simulink model "LQGdesign"  (R2019b)
settings: Solver=VariableStepAuto  StartTime=0.0  StopTime=3  RelTol=1e-3
values from neighbouring files (symbols this model uses):
  F2 = a*mass*g/(a+b)    (= 14.8072837402)    [main.m]
  g = 9.8    [EOM.m]    (also in main.m = 9.81)
  h0 = geometry_parameters(3)    [CalculateLoadCapacity.m]    (also in initialiseradialgap.m; main.m = 5e-05)
  Klqgi = lqr(Aaug,Baug,Qaug,Raug)    [main.m]
  Kps = (Vmax-Vmin)/(Hmax-Hmin)    (= 1666.66666667)    [main.m]
  Ksv = 30    [main.m]
  syskfd = c2d(syskf,Ts)    [main.m]
  tau = 0.12    [main.m]
  taus = 0.00125    [main.m]
  Ts = 1/fs    (= 0.001)    [main.m]
  xeq = x(end,1)    [main.m]
  yeq = x(end,3)    [main.m]
undefined symbols (not defined in the file or in its folder): DiscIntNeverNeededParam
libraries: neural x106, simulink x2
(part 1 of 3)
settings Model: Creator=Alexander  LastModifiedBy=Alexander

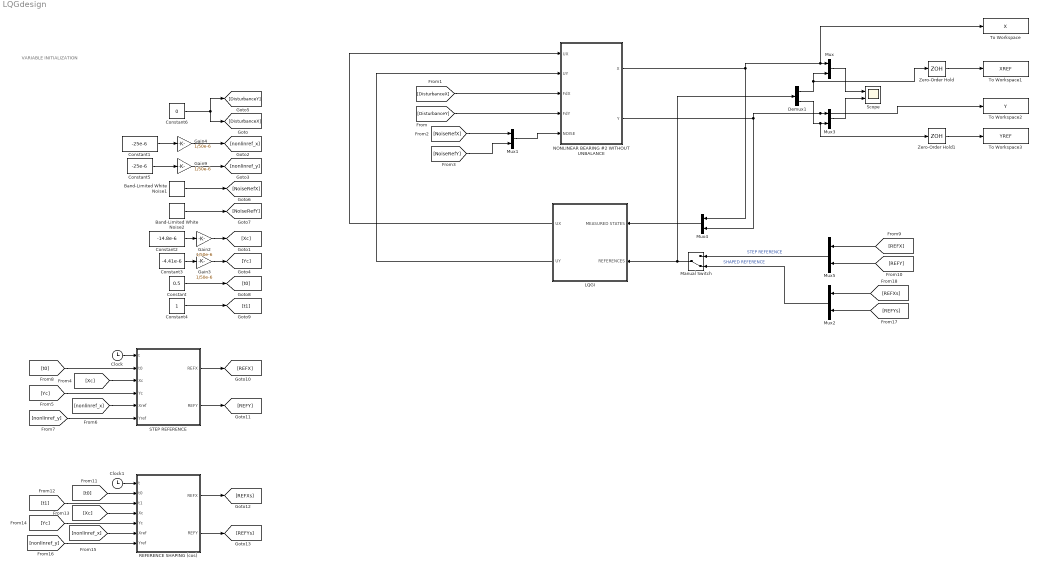
== system LQGdesign ==
  note: VARIABLE INITIALIZATION
  Band-Limited White Noise1 : simulink/Sources/Band-Limited White Noise  Cov=n_pow  Ts=Ts  seed=[23341]
  Band-Limited White Noise2 : simulink/Sources/Band-Limited White Noise  Cov=n_pow  Ts=1.1*Ts  seed=[23341]
  Clock : Clock
  Clock1 : Clock
  Constant : Constant  Value=0.5
  Constant1 : Constant  Value=-25e-6
  Constant2 : Constant  Value=-14.8e-6
  Constant3 : Constant  Value=-4.41e-6
  Constant4 : Constant
  Constant5 : Constant  Value=-25e-6
  Constant6 : Constant  Value=0
  Demux1 : Demux  Outputs=2
  Gain{2..4,9} (4 alike) : Gain  Gain=1/50e-6
  LQGI : Subsystem
  Manual Switch : ManualSwitch  CurrentSetting=0
  Mux{,1..5} (6 alike) : Mux  Inputs=2
  NONLINEAR BEARING #2 WITHOUT UNBALANCE : Subsystem
  REFERENCE SHAPING (cos) : MATLAB Function  TreatAsAtomicUnit=on
  STEP REFERENCE : MATLAB Function  TreatAsAtomicUnit=on
  Scope : Scope  NumInputPorts=2
  To Workspace : ToWorkspace  VariableName=X  SampleTime=-1
      settings: Save2DSignal=2-D array (concatenate along first dimension)
  To Workspace1 : ToWorkspace  VariableName=XREF  SampleTime=-1
      settings: Save2DSignal=2-D array (concatenate along first dimension)
  To Workspace2 : ToWorkspace  VariableName=Y  SampleTime=-1
      settings: Save2DSignal=2-D array (concatenate along first dimension)
  To Workspace3 : ToWorkspace  VariableName=YREF  SampleTime=-1
      settings: Save2DSignal=2-D array (concatenate along first dimension)
  Zero-Order Hold : ZeroOrderHold  SampleTime=Ts
  Zero-Order Hold1 : ZeroOrderHold  SampleTime=Ts
  wires:
  [nonlinref_x] -> STEP REFERENCE/5(Xref)
  Constant4/1 -> [t1]
  [NoiseRefY] -> Mux1/2
  Constant/1 -> [t0]
  [t0] -> STEP REFERENCE/2(t0)
  Clock/1 -> STEP REFERENCE/1(t)
  NONLINEAR BEARING #2 WITHOUT UNBALANCE/1(X) -> To Workspace/1, Mux/1, Mux4/1
  STEP REFERENCE/2(REFY) -> [REFY]
  Gain9/1 -> [nonlinref_y]
  Constant3/1 -> Gain3/1
  [Xc] -> STEP REFERENCE/3(Xc)
  [DisturbanceY] -> NONLINEAR BEARING #2 WITHOUT UNBALANCE/4(FdY)
  Mux3/1 -> Scope/2
  Gain3/1 -> [Yc]
  Gain2/1 -> [Xc]
  [DisturbanceX] -> NONLINEAR BEARING #2 WITHOUT UNBALANCE/3(FdX)
  NONLINEAR BEARING #2 WITHOUT UNBALANCE/2(Y) -> To Workspace2/1, Mux3/1, Mux4/2
  Constant5/1 -> Gain9/1
  STEP REFERENCE/1(REFX) -> [REFX]
  Demux1/1 -> Mux/2, Zero-Order Hold/1
  Gain4/1 -> [nonlinref_x]
  Mux2/1 -> Manual Switch/2  "SHAPED REFERENCE"
  REFERENCE SHAPING (cos)/1(REFX) -> [REFXs]
  Mux5/1 -> Manual Switch/1  "STEP REFERENCE"
  [Yc] -> STEP REFERENCE/4(Yc)
  [REFY] -> Mux5/2
  [REFXs] -> Mux2/1
  Mux/1 -> Scope/1
  [REFX] -> Mux5/1
  Constant2/1 -> Gain2/1
  [REFYs] -> Mux2/2
  Band-Limited White Noise1/1 -> [NoiseRefX]
  Demux1/2 -> Zero-Order Hold1/1, Mux3/2
  Mux1/1 -> NONLINEAR BEARING #2 WITHOUT UNBALANCE/5(NOISE)
  Clock1/1 -> REFERENCE SHAPING (cos)/1(t)
  [nonlinref_y] -> STEP REFERENCE/6(Yref)
  [nonlinref_x] -> REFERENCE SHAPING (cos)/6(Xref)
  Band-Limited White Noise2/1 -> [NoiseRefY]
  REFERENCE SHAPING (cos)/2(REFY) -> [REFYs]
  [Yc] -> REFERENCE SHAPING (cos)/5(Yc)
  [nonlinref_y] -> REFERENCE SHAPING (cos)/7(Yref)
  [Xc] -> REFERENCE SHAPING (cos)/4(Xc)
  Constant1/1 -> Gain4/1
  [t0] -> REFERENCE SHAPING (cos)/2(t0)
  [t1] -> REFERENCE SHAPING (cos)/3(t1)
  [NoiseRefX] -> Mux1/1
  Zero-Order Hold/1 -> To Workspace1/1
  Zero-Order Hold1/1 -> To Workspace3/1
  Constant6/1 -> [DisturbanceX], [DisturbanceY]
  Manual Switch/1 -> Demux1/1, LQGI/2(REFERENCES)
  LQGI/2("UY ") -> NONLINEAR BEARING #2 WITHOUT UNBALANCE/2(UY)
  LQGI/1(UX) -> NONLINEAR BEARING #2 WITHOUT UNBALANCE/1(UX)
  Mux4/1 -> LQGI/1(MEASURED STATES)

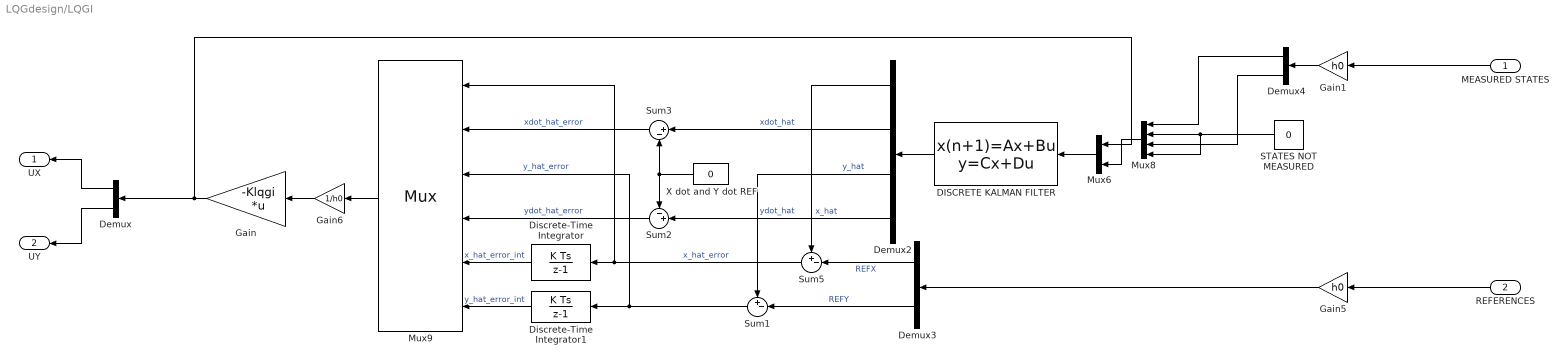
== system LQGdesign/LQGI ==
  MEASURED STATES : Inport
  REFERENCES : Inport  Port=2
  DISCRETE KALMAN FILTER : DiscreteStateSpace  A=syskfd.A  B=syskfd.B  C=syskfd.C  D=syskfd.D  SampleTime=Ts
  Demux : Demux  Outputs=2
  Demux2 : Demux
  Demux3 : Demux  Outputs=2
  Demux4 : Demux  Outputs=2
  Discrete-Time Integrator : DiscreteIntegrator  SampleTime=Ts  ICPrevOutput=DiscIntNeverNeededParam  ICPrevScaledInput=DiscIntNeverNeededParam
  Discrete-Time Integrator1 : DiscreteIntegrator  SampleTime=Ts  ICPrevOutput=DiscIntNeverNeededParam  ICPrevScaledInput=DiscIntNeverNeededParam
  Gain : Gain  Gain=-Klqgi  Multiplication=Matrix(K*u) (u vector)
  Gain1 : Gain  Gain=h0
  Gain5 : Gain  Gain=h0
  Gain6 : Gain  Gain=1/h0
  Mux6 : Mux  Inputs=2
  Mux8 : Mux
  Mux9 : Mux  Inputs=6
      settings: DisplayOption=signals
  STATES NOT MEASURED : Constant  Value=0
  Sum1 : Sum  Inputs=+-|
  Sum2 : Sum  Inputs=-+|
  Sum3 : Sum  Inputs=|+-
  Sum5 : Sum  Inputs=+-|
  X dot and Y dot REF : Constant  Value=0
  UX : Outport
  "UY " : Outport  Port=2
  wires:
  Demux2/1 -> Sum5/1  "x_hat"
  Gain6/1 -> Gain/1
  Mux6/1 -> DISCRETE KALMAN FILTER/1
  Discrete-Time Integrator1/1 -> Mux9/6  "y_hat_error_int"
  Demux4/1 -> Mux8/1
  DISCRETE KALMAN FILTER/1 -> Demux2/1
  Demux3/1 -> Sum5/2  "REFX"
  Gain1/1 -> Demux4/1
  Gain/1 -> Mux6/1, Demux/1
  Mux9/1 -> Gain6/1
  Sum1/1 -> Discrete-Time Integrator1/1, Mux9/3  "y_hat_error"
  MEASURED STATES/1 -> Gain1/1
  Mux8/1 -> Mux6/2
  STATES NOT MEASURED/1 -> Mux8/4, Mux8/2
  Demux4/2 -> Mux8/3
  Sum3/1 -> Mux9/2  "xdot_hat_error"
  Demux/1 -> UX/1
  Discrete-Time Integrator/1 -> Mux9/5  "x_hat_error_int"
  Sum5/1 -> Discrete-Time Integrator/1, Mux9/1  "x_hat_error"
  Demux2/2 -> Sum3/1  "xdot_hat"
  X dot and Y dot REF/1 -> Sum2/1, Sum3/2
  Demux3/2 -> Sum1/2  "REFY"
  Sum2/1 -> Mux9/4  "ydot_hat_error"
  Demux2/3 -> Sum1/1  "y_hat"
  Demux2/4 -> Sum2/2  "ydot_hat"
  Gain5/1 -> Demux3/1
  Demux/2 -> "UY "/1
  REFERENCES/1 -> Gain5/1

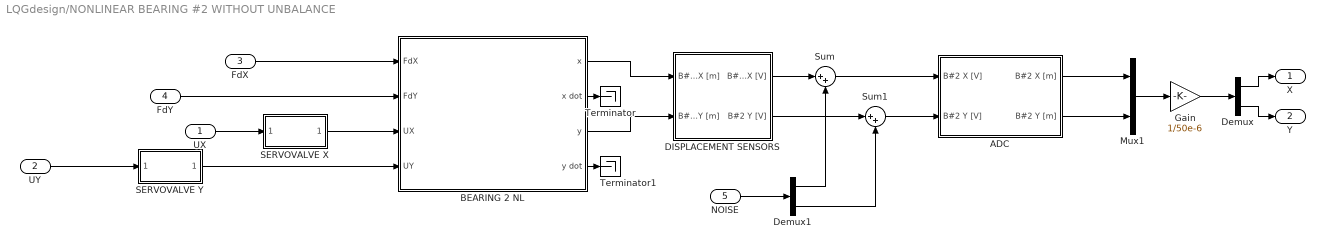
== system LQGdesign/NONLINEAR BEARING #2 WITHOUT UNBALANCE ==
  UX : Inport
  UY : Inport  Port=2
  FdX : Inport  Port=3
  FdY : Inport  Port=4
  NOISE : Inport  Port=5
  ADC : Subsystem
  BEARING 2 NL : Subsystem
  DISPLACEMENT SENSORS : Subsystem
  Demux : Demux  Outputs=2
  Demux1 : Demux  Outputs=2
  Gain : Gain  Gain=1/50e-6
  Mux1 : Mux  Inputs=2
  SERVOVALVE X : Subsystem
  SERVOVALVE Y : Subsystem
  Sum : Sum  Inputs=|++
  Sum1 : Sum  Inputs=|++
  Terminator : Terminator
  Terminator1 : Terminator
  X : Outport
  Y : Outport  Port=2
  wires:
  ADC/2(B#2 Y [m]) -> Mux1/2
  ADC/1(B#2 X [m]) -> Mux1/1
  Mux1/1 -> Gain/1
  Demux/1 -> X/1
  Gain/1 -> Demux/1
  Demux/2 -> Y/1
  BEARING 2 NL/3(y) -> DISPLACEMENT SENSORS/2(B#2 Y [m])
  BEARING 2 NL/1(x) -> DISPLACEMENT SENSORS/1(B#2 X [m])
  Demux1/2 -> Sum1/2
  NOISE/1 -> Demux1/1
  Demux1/1 -> Sum/2
  Sum1/1 -> ADC/2(B#2 Y [V])
  Sum/1 -> ADC/1(B#2 X [V])
  DISPLACEMENT SENSORS/1(B#2 X [V]) -> Sum/1
  DISPLACEMENT SENSORS/2(B#2 Y [V]) -> Sum1/1
  BEARING 2 NL/4(y dot) -> Terminator1/1
  BEARING 2 NL/2("x dot ") -> Terminator/1
  FdX/1 -> BEARING 2 NL/1(FdX)
  UX/1 -> SERVOVALVE X/1(Uv [V])
  SERVOVALVE Y/1(Uf [F]) -> BEARING 2 NL/4(UY)
  UY/1 -> SERVOVALVE Y/1(Uv [V])
  FdY/1 -> BEARING 2 NL/2(FdY)
  SERVOVALVE X/1(Uf [F]) -> BEARING 2 NL/3(UX)

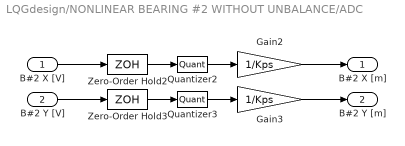
== system LQGdesign/NONLINEAR BEARING #2 WITHOUT UNBALANCE/ADC ==
  B#2 X [V] : Inport
  B#2 Y [V] : Inport  Port=2
  Gain2 : Gain  Gain=1/Kps
  Gain3 : Gain  Gain=1/Kps
  Quantizer2 : Quantizer  QuantizationInterval=0.000152587890625
  Quantizer3 : Quantizer  QuantizationInterval=0.000152587890625
  Zero-Order Hold2 : ZeroOrderHold  SampleTime=Ts
  Zero-Order Hold3 : ZeroOrderHold  SampleTime=Ts
  B#2 X [m] : Outport
  B#2 Y [m] : Outport  Port=2
  wires:
  B#2 Y [V]/1 -> Zero-Order Hold3/1
  Zero-Order Hold3/1 -> Quantizer3/1
  Gain3/1 -> B#2 Y [m]/1
  Zero-Order Hold2/1 -> Quantizer2/1
  Gain2/1 -> B#2 X [m]/1
  B#2 X [V]/1 -> Zero-Order Hold2/1
  Quantizer3/1 -> Gain3/1
  Quantizer2/1 -> Gain2/1

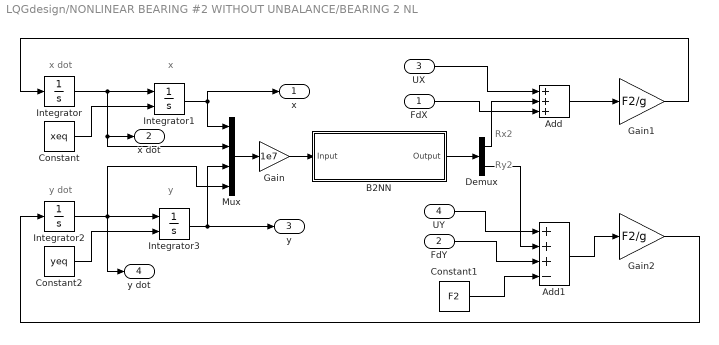
== system LQGdesign/NONLINEAR BEARING #2 WITHOUT UNBALANCE/BEARING 2 NL ==
  note: x
  note: x dot
  note: y
  note: y dot
  note: Ry2
  note: Rx2
  FdX : Inport
  FdY : Inport  Port=2
  UX : Inport  Port=3
  UY : Inport  Port=4
  Add : Sum  Inputs=+++
  Add1 : Sum  Inputs=+++-
  B2NN : Subsystem
      mask help: Feed-Forward Neural Network
      mask Display: fprintf('BEARING #2 NN');port_label('input',1,' X');port_label('output',1,'F');
  Constant : Constant  Value=xeq
  Constant1 : Constant  Value=F2
  Constant2 : Constant  Value=yeq
  Demux : Demux  Outputs=2
  Gain : Gain  Gain=1e7
  Gain1 : Gain  Gain=F2/g
  Gain2 : Gain  Gain=F2/g
  Integrator : Integrator
  Integrator1 : Integrator  InitialConditionSource=external
  Integrator2 : Integrator
  Integrator3 : Integrator  InitialConditionSource=external
  Mux : Mux
  x : Outport
  "x dot " : Outport  Port=2
  y : Outport  Port=3
  y dot : Outport  Port=4
  wires:
  Add1/1 -> Gain2/1
  Gain1/1 -> Integrator/1
  FdY/1 -> Add1/3
  Integrator/1 -> "x dot "/1, Mux/2, Integrator1/1
  Integrator1/1 -> x/1, Mux/1
  Integrator2/1 -> y dot/1, Mux/4, Integrator3/1
  Add/1 -> Gain1/1
  Integrator3/1 -> y/1, Mux/3
  FdX/1 -> Add/3
  Mux/1 -> Gain/1
  Demux/2 -> Add1/2
  Gain/1 -> B2NN/1(Input)
  Demux/1 -> Add/2
  Gain2/1 -> Integrator2/1
  Constant1/1 -> Add1/4
  B2NN/1(Output) -> Demux/1
  UX/1 -> Add/1
  UY/1 -> Add1/1
  Constant/1 -> Integrator1/2
  Constant2/1 -> Integrator3/2

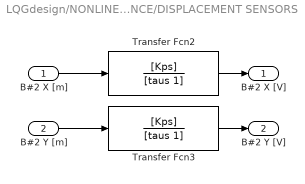
== system LQGdesign/NONLINEAR BEARING #2 WITHOUT UNBALANCE/DISPLACEMENT SENSORS ==
  B#2 X [m] : Inport
  B#2 Y [m] : Inport  Port=2
  Transfer Fcn2 : TransferFcn  Numerator=[Kps]  Denominator=[taus 1]
  Transfer Fcn3 : TransferFcn  Numerator=[Kps]  Denominator=[taus 1]
  B#2 X [V] : Outport
  B#2 Y [V] : Outport  Port=2
  wires:
  Transfer Fcn3/1 -> B#2 Y [V]/1
  Transfer Fcn2/1 -> B#2 X [V]/1
  B#2 X [m]/1 -> Transfer Fcn2/1
  B#2 Y [m]/1 -> Transfer Fcn3/1

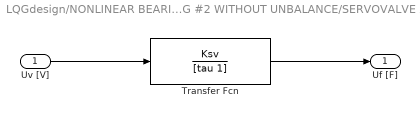
== system LQGdesign/NONLINEAR BEARING #2 WITHOUT UNBALANCE/SERVOVALVE X ==
  Uv [V] : Inport
  Transfer Fcn : TransferFcn  Numerator=Ksv  Denominator=[tau 1]
  Uf [F] : Outport
  wires:
  Uv [V]/1 -> Transfer Fcn/1
  Transfer Fcn/1 -> Uf [F]/1

== system LQGdesign/NONLINEAR BEARING #2 WITHOUT UNBALANCE/SERVOVALVE Y ==
  Uv [V] : Inport
  Transfer Fcn : TransferFcn  Numerator=Ksv  Denominator=[tau 1]
  Uf [F] : Outport
  wires:
  Transfer Fcn/1 -> Uf [F]/1
  Uv [V]/1 -> Transfer Fcn/1

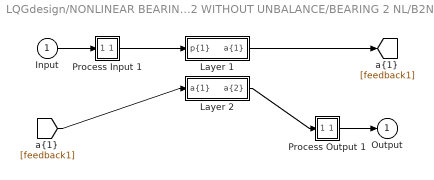
== system LQGdesign/NONLINEAR BEARING #2 WITHOUT UNBALANCE/BEARING 2 NL/B2NN ==
  Input : Inport  PortDimensions=4
      mask Display: e = 0.06;c1 = [120 230 180]/255;c2 = ([120 230 180]+0)/(256+128);c3 = ([120 230 180]+128)/(256+128);patch([0 1 1 0],[0 0 1 1],c1);patch([0 1 1 1-e 1-e 0+e],[0 0 1 1-e 0+e 0+e],c2);patch([0 0 1 1-e 0+e 0+e],[0 1 1 1-e 1-e 0+e],c3);plot([0 1 1 0 0],[0 0 1 1 0]);
  Layer 1 : Subsystem
      mask Display: e = 0.06;c1 = [120 150 230]/255;c2 = ([120 150 230]+0)/383;c3 = ([120 150 230]+128)/383;patch([0 1 1 0],[0 0 1 1],c1);patch([0 1 1 1-e 1-e 0+e],[0 0 1 1-e 0+e 0+e],c2);patch([0 0 1 1-e 0+e 0+e],[0 1 1 1-e 1-e 0+e],c3);plot([0 1 1 0 0],[0 0 1 1 0]);
  Layer 2 : Subsystem
      mask Display: e = 0.06;c1 = [120 150 230]/255;c2 = ([120 150 230]+0)/383;c3 = ([120 150 230]+128)/383;patch([0 1 1 0],[0 0 1 1],c1);patch([0 1 1 1-e 1-e 0+e],[0 0 1 1-e 0+e 0+e],c2);patch([0 0 1 1-e 0+e 0+e],[0 1 1 1-e 1-e 0+e],c3);plot([0 1 1 0 0],[0 0 1 1 0]);
  Process Input 1 : Subsystem
      mask Display: e = 0.06;c1 = [120 150 230]/255;c2 = ([120 150 230]+0)/383;c3 = ([120 150 230]+128)/383;patch([0 1 1 0],[0 0 1 1],c1);patch([0 1 1 1-e 1-e 0+e],[0 0 1 1-e 0+e 0+e],c2);patch([0 0 1 1-e 0+e 0+e],[0 1 1 1-e 1-e 0+e],c3);plot([0 1 1 0 0],[0 0 1 1 0]);
  Process Output 1 : Subsystem
      mask Display: e = 0.06;c1 = [120 150 230]/255;c2 = ([120 150 230]+0)/383;c3 = ([120 150 230]+128)/383;patch([0 1 1 0],[0 0 1 1],c1);patch([0 1 1 1-e 1-e 0+e],[0 0 1 1-e 0+e 0+e],c2);patch([0 0 1 1-e 0+e 0+e],[0 1 1 1-e 1-e 0+e],c3);plot([0 1 1 0 0],[0 0 1 1 0]);
  Output : Outport  InitialOutput=[0;0]
      mask Display: e = 0.06;c1 = [120 230 180]/255;c2 = ([120 230 180]+0)/(256+128);c3 = ([120 230 180]+128)/(256+128);patch([0 1 1 0],[0 0 1 1],c1);patch([0 1 1 1-e 1-e 0+e],[0 0 1 1-e 0+e 0+e],c2);patch([0 0 1 1-e 0+e 0+e],[0 1 1 1-e 1-e 0+e],c3);plot([0 1 1 0 0],[0 0 1 1 0]);
  wires:
  Input/1 -> Process Input 1/1(x)
  Process Output 1/1(y) -> Output/1
  Process Input 1/1(p) -> Layer 1/1("p{1}")
  Layer 1/1("a{1}") -> [feedback1]
  [feedback1] -> Layer 2/1("a{1} ")
  Layer 2/1("a{2}") -> Process Output 1/1(a)

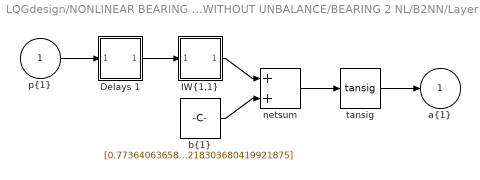
== system LQGdesign/NONLINEAR BEARING #2 WITHOUT UNBALANCE/BEARING 2 NL/B2NN/Layer 1 ==
  "p{1}" : Inport  PortDimensions=4
      mask Display: e = 0.06;c1 = [120 230 180]/255;c2 = ([120 230 180]+0)/(256+128);c3 = ([120 230 180]+128)/(256+128);patch([0 1 1 0],[0 0 1 1],c1);patch([0 1 1 1-e 1-e 0+e],[0 0 1 1-e 0+e 0+e],c2);patch([0 0 1 1-e 0+e 0+e],[0 1 1 1-e 1-e 0+e],c3);plot([0 1 1 0 0],[0 0 1 1 0]);
  Delays 1 : Subsystem
      mask Display: e = 0.06;c1 = [120 150 230]/255;c2 = ([120 150 230]+0)/383;c3 = ([120 150 230]+128)/383;patch([0 1 1 0],[0 0 1 1],c1);patch([0 1 1 1-e 1-e 0+e],[0 0 1 1-e 0+e 0+e],c2);patch([0 0 1 1-e 0+e 0+e],[0 1 1 1-e 1-e 0+e],c3);plot([0 1 1 0 0],[0 0 1 1 0]);disp('0');
  "IW{1,1}" : Subsystem
      mask Display: e = 0.06;c1 = [120 150 230]/255;c2 = ([120 150 230]+0)/383;c3 = ([120 150 230]+128)/383;patch([0 1 1 0],[0 0 1 1],c1);patch([0 1 1 1-e 1-e 0+e],[0 0 1 1-e 0+e 0+e],c2);patch([0 0 1 1-e 0+e 0+e],[0 1 1 1-e 1-e 0+e],c3);plot([0 1 1 0 0],[0 0 1 1 0]);disp('W');
  "b{1}" : Constant  Value=[0.77364063658353299235415079238009639084339141845703125;-0.5742401500824383386856197830638848245143890380859375;2.18924884343246173301622548024170100688934326171875;0.7247679770582233782505454655620269477367401123046875;1.50920298605198599517507318523712456226348876953125;0.2251254120036607908605930106205050833523273468017578125;1.31581849386470395302239921875298023223876953125;-1.4439178611363931992173093021847307682037353515625;-0.6388738634319419684715057883295230567455291748046875;0.42713022702700664812169861761503852903842926025390625;-5.50585208820272331564638079726137220859527587890625;1.0116121407127753872856601446983404457569122314453125;0.1855740272752877950690475472583784721791744232177734375;-2.752365697458559079535689306794665753841400146484375;-5.11790555901796029303341128979809582233428955078125;-0.338655420078370517078525381293729878962039947509765625;1.1393557433472689677245170969399623572826385498046875;-2.759792246021837147651467603282071650028228759765625;0.397902004749398463534504344352171756327152252197265625;3.409108583987378704449611177551560103893280029296875;0.5735207395663535212548822528333403170108795166015625;6.01140115256299356616409568232484161853790283203125;1.7685521361064504564097887850948609411716461181640625;-0.340503549829671514626028283601044677197933197021484375;3.014660128394303750809513076092116534709930419921875;5.29104737030530003494277480058372020721435546875;1.8018829599315646650126154781901277601718902587890625;-3.780494805335994801254173580673523247241973876953125;-0.82794048304963963058611398082575760781764984130859375;-0.75276220003998017826774002969614230096340179443359375;-0.918260179670823628583775644074194133281707763671875;-1.5960749465646273392849252559244632720947265625;2.280202799305620420255991120939143002033233642578125;0.6798608356003492669827892314060591161251068115234375;0.00037235437068993369746916499707367620430886745452880859375;0.337122632082677398113190747608314268290996551513671875;-1.3454473348402427035352957318536937236785888671875;0.01443955672754803666590905919520082534290850162506103515625;-0.1776195368516353401133756051422096788883209228515625;1.4978387755899638111856120303855277597904205322265625;1.46539531018312541021941797225736081600189208984375;-0.32071205937207902803010028947028331458568572998046875;-1.90744419520537444867613885435275733470916748046875;-11.9891606982089005128955250256694853305816650390625;-2.1669887121737634316787080024369060993194580078125;0.3672127830607030407605861910269595682621002197265625;-0.06203580478551275201315462481943541206419467926025390625;-2.93472369606861160917787856305949389934539794921875;1.75388849018205572605211273184977471828460693359375;0.697291453036331443371409477549605071544647216796875;-0.0645312657524038379985853453035815618932247161865234375;3.764184402430989617727163931704126298427581787109375;1.7961663654062818284984359706868417561054229736328125;-0.8081845398239464461909165038377977907657623291015625;0.78181635523739334558968039345927536487579345703125;-4.5319131193828585679739262559451162815093994140625;0.024789841792795141994787400108180008828639984130859375;-6.117333706507910306982012116350233554840087890625;-1.52321329303906960461745256907306611537933349609375;-0.6842591181818225010147216380573809146881103515625;0.656524530984853083026564490864984691143035888671875;-0.724499291455265481687320061610080301761627197265625;2.936003111628732842319777773809619247913360595703125;-0.87591317415541547486412810030742548406124114990234375;-5.40320016731756869177161206607706844806671142578125;-0.08928640781480877419706843056701472960412502288818359375;2.76745317279060021320447049220092594623565673828125;-0.36100903729607425329817260717391036450862884521484375;-0.2338154075428852951556990547032910399138927459716796875;5.617788840059471766608112375251948833465576171875;-0.18177176297821329153947544909897260367870330810546875;-2.897641100484706466744455610751174390316009521484375 ...(+1531 chars)]
      mask Display: e = 0.06;c1 = [120 150 230]/255;c2 = ([120 150 230]+0)/383;c3 = ([120 150 230]+128)/383;patch([0 1 1 0],[0 0 1 1],c1);patch([0 1 1 1-e 1-e 0+e],[0 0 1 1-e 0+e 0+e],c2);patch([0 0 1 1-e 0+e 0+e],[0 1 1 1-e 1-e 0+e],c3);plot([0 1 1 0 0],[0 0 1 1 0]);disp('b');
  netsum : Sum  Inputs=2  SaturateOnIntegerOverflow=on  InputSameDT=on  OutDataTypeStr=Inherit: Same as first input
      mask Display: e = 0.06;c1 = [120 150 230]/255;c2 = ([120 150 230]+0)/383;c3 = ([120 150 230]+128)/383;patch([0 1 1 0],[0 0 1 1],c1);patch([0 1 1 1-e 1-e 0+e],[0 0 1 1-e 0+e 0+e],c2);patch([0 0 1 1-e 0+e 0+e],[0 1 1 1-e 1-e 0+e],c3);plot([0 1 1 0 0],[0 0 1 1 0]);disp('+');
  tansig : neural/Transfer Functions/tansig
      settings: SourceProductName=Deep Learning Toolbox
  "a{1}" : Outport  InitialOutput=[0;0;0;0;0;0;0;0;0;0;0;0;0;0;0;0;0;0;0;0;0;0;0;0;0;0;0;0;0;0;0;0;0;0;0;0;0;0;0;0;0;0;0;0;0;0;0;0;0;0;0;0;0;0;0;0;0;0;0;0;0;0;0;0;0;0;0;0;0;0;0;0;0;0;0;0;0;0;0;0;0;0;0;0;0;0;0;0;0;0;0;0;0;0;0;0;0;0;0;0]
      mask Display: e = 0.06;c1 = [120 230 180]/255;c2 = ([120 230 180]+0)/(256+128);c3 = ([120 230 180]+128)/(256+128);patch([0 1 1 0],[0 0 1 1],c1);patch([0 1 1 1-e 1-e 0+e],[0 0 1 1-e 0+e 0+e],c2);patch([0 0 1 1-e 0+e 0+e],[0 1 1 1-e 1-e 0+e],c3);plot([0 1 1 0 0],[0 0 1 1 0]);
  wires:
  "p{1}"/1 -> Delays 1/1("p{1}")
  Delays 1/1("pd{1,1}") -> "IW{1,1}"/1("pd{1,1}")
  "IW{1,1}"/1("iz{1,1}") -> netsum/1
  "b{1}"/1 -> netsum/2
  netsum/1 -> tansig/1
  tansig/1 -> "a{1}"/1

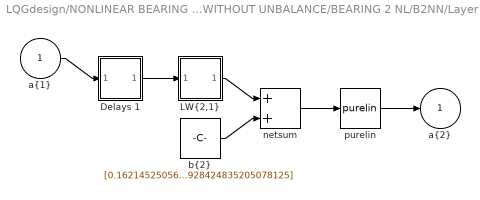
== system LQGdesign/NONLINEAR BEARING #2 WITHOUT UNBALANCE/BEARING 2 NL/B2NN/Layer 2 ==
  "a{1} " : Inport  PortDimensions=100
      mask Display: e = 0.06;c1 = [120 230 180]/255;c2 = ([120 230 180]+0)/(256+128);c3 = ([120 230 180]+128)/(256+128);patch([0 1 1 0],[0 0 1 1],c1);patch([0 1 1 1-e 1-e 0+e],[0 0 1 1-e 0+e 0+e],c2);patch([0 0 1 1-e 0+e 0+e],[0 1 1 1-e 1-e 0+e],c3);plot([0 1 1 0 0],[0 0 1 1 0]);
  Delays 1 : Subsystem
      mask Display: e = 0.06;c1 = [120 150 230]/255;c2 = ([120 150 230]+0)/383;c3 = ([120 150 230]+128)/383;patch([0 1 1 0],[0 0 1 1],c1);patch([0 1 1 1-e 1-e 0+e],[0 0 1 1-e 0+e 0+e],c2);patch([0 0 1 1-e 0+e 0+e],[0 1 1 1-e 1-e 0+e],c3);plot([0 1 1 0 0],[0 0 1 1 0]);disp('0');
  "LW{2,1}" : Subsystem
      mask Display: e = 0.06;c1 = [120 150 230]/255;c2 = ([120 150 230]+0)/383;c3 = ([120 150 230]+128)/383;patch([0 1 1 0],[0 0 1 1],c1);patch([0 1 1 1-e 1-e 0+e],[0 0 1 1-e 0+e 0+e],c2);patch([0 0 1 1-e 0+e 0+e],[0 1 1 1-e 1-e 0+e],c3);plot([0 1 1 0 0],[0 0 1 1 0]);disp('W');
  "b{2}" : Constant  Value=[0.162145250569083076985776870060362853109836578369140625;3.253717818452451115973644846235401928424835205078125]
      mask Display: e = 0.06;c1 = [120 150 230]/255;c2 = ([120 150 230]+0)/383;c3 = ([120 150 230]+128)/383;patch([0 1 1 0],[0 0 1 1],c1);patch([0 1 1 1-e 1-e 0+e],[0 0 1 1-e 0+e 0+e],c2);patch([0 0 1 1-e 0+e 0+e],[0 1 1 1-e 1-e 0+e],c3);plot([0 1 1 0 0],[0 0 1 1 0]);disp('b');
  netsum : Sum  Inputs=2  SaturateOnIntegerOverflow=on  InputSameDT=on  OutDataTypeStr=Inherit: Same as first input
      mask Display: e = 0.06;c1 = [120 150 230]/255;c2 = ([120 150 230]+0)/383;c3 = ([120 150 230]+128)/383;patch([0 1 1 0],[0 0 1 1],c1);patch([0 1 1 1-e 1-e 0+e],[0 0 1 1-e 0+e 0+e],c2);patch([0 0 1 1-e 0+e 0+e],[0 1 1 1-e 1-e 0+e],c3);plot([0 1 1 0 0],[0 0 1 1 0]);disp('+');
  purelin : neural/Transfer Functions/purelin
      settings: SourceProductName=Deep Learning Toolbox
  "a{2}" : Outport  InitialOutput=[0;0]
      mask Display: e = 0.06;c1 = [120 230 180]/255;c2 = ([120 230 180]+0)/(256+128);c3 = ([120 230 180]+128)/(256+128);patch([0 1 1 0],[0 0 1 1],c1);patch([0 1 1 1-e 1-e 0+e],[0 0 1 1-e 0+e 0+e],c2);patch([0 0 1 1-e 0+e 0+e],[0 1 1 1-e 1-e 0+e],c3);plot([0 1 1 0 0],[0 0 1 1 0]);
  wires:
  "a{1} "/1 -> Delays 1/1("p{2}")
  Delays 1/1("pd{2,1}") -> "LW{2,1}"/1("ad{2,1}")
  "LW{2,1}"/1("lz{2,1}") -> netsum/1
  "b{2}"/1 -> netsum/2
  netsum/1 -> purelin/1
  purelin/1 -> "a{2}"/1

== system LQGdesign/NONLINEAR BEARING #2 WITHOUT UNBALANCE/BEARING 2 NL/B2NN/Process Input 1 ==
  x : Inport  PortDimensions=4
      mask Display: e = 0.06;c1 = [120 230 180]/255;c2 = ([120 230 180]+0)/(256+128);c3 = ([120 230 180]+128)/(256+128);patch([0 1 1 0],[0 0 1 1],c1);patch([0 1 1 1-e 1-e 0+e],[0 0 1 1-e 0+e 0+e],c2);patch([0 0 1 1-e 0+e 0+e],[0 1 1 1-e 1-e 0+e],c3);plot([0 1 1 0 0],[0 0 1 1 0]);
  mapminmax : neural/Processing Functions/mapminmax  xmin=[-416.751800229438060796383069828;-77252.7627451588050462305545807;-412.604732780781148449023021385;-87738.2155925167608074843883514]  xmax=[420.767069573879723520803963766;77306.0606816288054687902331352;399.854305951324249690514989197;66574.8201504489697981625795364]  ymin=-1  ymax=1
      settings: SourceProductName=Deep Learning Toolbox
  p : Outport  PortDimensions=4
      mask Display: e = 0.06;c1 = [120 230 180]/255;c2 = ([120 230 180]+0)/(256+128);c3 = ([120 230 180]+128)/(256+128);patch([0 1 1 0],[0 0 1 1],c1);patch([0 1 1 1-e 1-e 0+e],[0 0 1 1-e 0+e 0+e],c2);patch([0 0 1 1-e 0+e 0+e],[0 1 1 1-e 1-e 0+e],c3);plot([0 1 1 0 0],[0 0 1 1 0]);
  wires:
  x/1 -> mapminmax/1
  mapminmax/1 -> p/1

== system LQGdesign/NONLINEAR BEARING #2 WITHOUT UNBALANCE/BEARING 2 NL/B2NN/Process Output 1 ==
  a : Inport  PortDimensions=2
      mask Display: e = 0.06;c1 = [120 230 180]/255;c2 = ([120 230 180]+0)/(256+128);c3 = ([120 230 180]+128)/(256+128);patch([0 1 1 0],[0 0 1 1],c1);patch([0 1 1 1-e 1-e 0+e],[0 0 1 1-e 0+e 0+e],c2);patch([0 0 1 1-e 0+e 0+e],[0 1 1 1-e 1-e 0+e],c3);plot([0 1 1 0 0],[0 0 1 1 0]);
  mapminmax_reverse : neural/Processing Functions/mapminmax_reverse  xmin=[-106.274577764110574662481667474;-90.0138039858543947957514319569]  xmax=[105.37554263525613862384489039;121.561184920492564742744434625]  ymin=-1  ymax=1
      settings: SourceProductName=Deep Learning Toolbox
  y : Outport  PortDimensions=2
      mask Display: e = 0.06;c1 = [120 230 180]/255;c2 = ([120 230 180]+0)/(256+128);c3 = ([120 230 180]+128)/(256+128);patch([0 1 1 0],[0 0 1 1],c1);patch([0 1 1 1-e 1-e 0+e],[0 0 1 1-e 0+e 0+e],c2);patch([0 0 1 1-e 0+e 0+e],[0 1 1 1-e 1-e 0+e],c3);plot([0 1 1 0 0],[0 0 1 1 0]);
  wires:
  a/1 -> mapminmax_reverse/1
  mapminmax_reverse/1 -> y/1

== system LQGdesign/NONLINEAR BEARING #2 WITHOUT UNBALANCE/BEARING 2 NL/B2NN/Layer 1/Delays 1 ==
  "p{1}" : Inport  PortDimensions=4
      mask Display: e = 0.06;c1 = [120 230 180]/255;c2 = ([120 230 180]+0)/(256+128);c3 = ([120 230 180]+128)/(256+128);patch([0 1 1 0],[0 0 1 1],c1);patch([0 1 1 1-e 1-e 0+e],[0 0 1 1-e 0+e 0+e],c2);patch([0 0 1 1-e 0+e 0+e],[0 1 1 1-e 1-e 0+e],c3);plot([0 1 1 0 0],[0 0 1 1 0]);
  mux : Mux  Inputs=1
      mask Display: e = 0.06;c1 = [120 150 230]/255;c2 = ([120 150 230]+0)/383;c3 = ([120 150 230]+128)/383;patch([0 1 1 0],[0 0 1 1],c1);patch([0 1 1 1-e 1-e 0+e],[0 0 1 1-e 0+e 0+e],c2);patch([0 0 1 1-e 0+e 0+e],[0 1 1 1-e 1-e 0+e],c3);plot([0 1 1 0 0],[0 0 1 1 0]);disp('Mux')
  "pd{1,1}" : Outport
      mask Display: e = 0.06;c1 = [120 230 180]/255;c2 = ([120 230 180]+0)/(256+128);c3 = ([120 230 180]+128)/(256+128);patch([0 1 1 0],[0 0 1 1],c1);patch([0 1 1 1-e 1-e 0+e],[0 0 1 1-e 0+e 0+e],c2);patch([0 0 1 1-e 0+e 0+e],[0 1 1 1-e 1-e 0+e],c3);plot([0 1 1 0 0],[0 0 1 1 0]);
  wires:
  "p{1}"/1 -> mux/1
  mux/1 -> "pd{1,1}"/1
